simulink model "RRplanar_sim"  (Simulink 7.1)
settings: Solver=ode45  StartTime=0.0  StopTime=10.0  RelTol=1e-3
libraries: roblocks x2
settings Model: Creator=Dario  LastModifiedBy=Dario

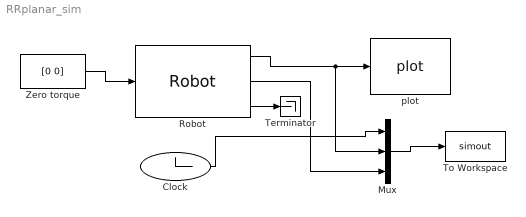
== system RRplanar_sim ==
  Clock : Clock
  Mux : Mux  Inputs=3
  Robot : roblocks/Robot  SystemSampleTime=-1  robot=RRplanar  q0=[0 0]
  Terminator : Terminator
  To Workspace : ToWorkspace  VariableName=simout  SampleTime=-1  SaveFormat=Array
  Zero torque : Constant  Value=[0 0]
  plot : roblocks/plot  SystemSampleTime=-1  robot=RRplanar
  wires:
  Robot/1 -> plot/1, Mux/2
  Zero torque/1 -> Robot/1
  Robot/3 -> Terminator/1
  Mux/1 -> To Workspace/1
  Robot/2 -> Mux/3
  Clock/1 -> Mux/1
